simulink library "stb"  (Simulink 8.1)
settings: Solver=ode1  StartTime=0.0  StopTime=Inf  FixedStep=0.001  RelTol=1e-3
PostLoadFcn:
  | , if any(exist('dsrtsu_mdlpostloadfcn', 'file') == [2, 3, 6]), try dsrtsu_mdlpostloadfcn('Execute', bdroot); catch fprintf('Error in PostLoadFcn (dsrtsu_mdlpostloadfcn) for model "%s":\n %s\n', bdroot, lasterr); end, end,
undefined symbols (not defined in the file or in its folder): KACC_ACCDecelReleaseMargin_kph, KACC_ACCDecelStartMargin_kph
libraries: hcu_lib x3
settings Model: DSRTSU_INTERNAL_RTI_VER=450  DSRTSU_INTERNAL_RTI_TYPE=rti1401  RTICANMMDATA=struct('GeneralSetupData',struct('modelroot','D:\ELN150201_TAIWAN\trunk\AdasDragon\software\sw_development\arch\app\acc','generalsettings',struct('filesettings',struct('destfolder',struct('Name','RTICANMM_FILES','Check',1),'buildfolder',struct('Name','.','Check',1),'AbsDestfolder',struct('Name','D:\ELN150201_TAIWAN\trunk\AdasDragon\software\sw_development\arch\app\acc\RTICANMM_FILES'),'AbsBuildfolder',struct('Name','D:\ELN150201_TAIWAN\trunk\AdasDragon\software\sw_development\arch\app\acc'))),'options',struct('addpaths',1,'rmpaths',1,'addtrcexclusion',logical(1),'cannavigator',struct('checkmonitoring',0),'show_usrtrc',0,'use_usrtrc',0),'advanced',struct('options',[1 1 1 1 1 1 1 1 1 1 1 1 1 1 1 1 1 1 1 1 1 1 1 1 1 1 1 1 1 1 1 1 1 1 1 1 1 1 1 1 1 1 1 1 1 1 1 1 1 1 1 1 1 1 1 1 1 1 1 1 1 1 1 1 1 1 1 1 1 1 1 1 1 1 1 1 1 1 1 1 1 1 1 1 1 1 1 1 1 1 1 1 1 1 1 1 1 1 1 1]),'MPSetup',{{}},'modelname','stb','block','stb'))  DSRTSU_INTERNAL_RTIFPGA=40  Creator=AT015555  LastModifiedBy=AT015555

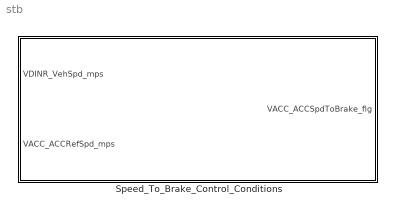
== system stb ==
  Speed_To_Brake_Control_Conditions : Subsystem

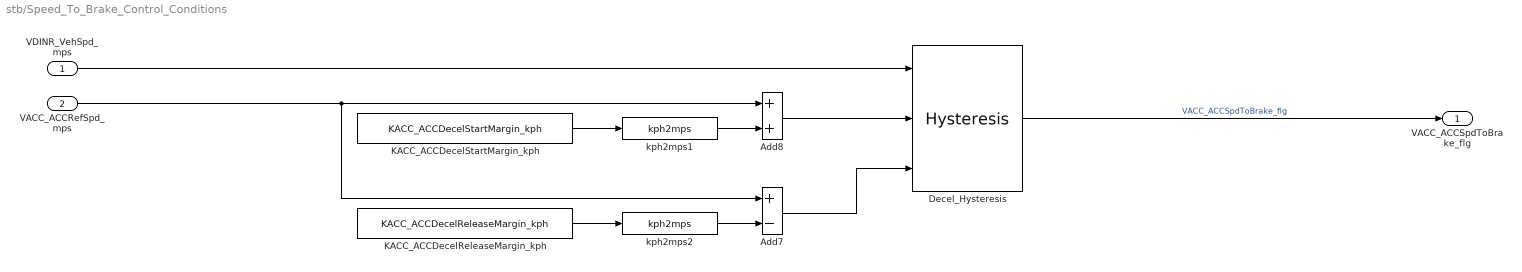
== system stb/Speed_To_Brake_Control_Conditions ==
  VDINR_VehSpd_mps : Inport
  VACC_ACCRefSpd_mps : Inport  Port=2
  Add7 : Sum  Inputs=+-
  Add8 : Sum
  Decel_Hysteresis : hcu_lib/Hysteresis  SystemSampleTime=-1
  KACC_ACCDecelReleaseMargin_kph : Constant  Value=KACC_ACCDecelReleaseMargin_kph  OutDataTypeStr=single
  KACC_ACCDecelStartMargin_kph : Constant  Value=KACC_ACCDecelStartMargin_kph  OutDataTypeStr=single
  kph2mps1 : hcu_lib/kph2mps
  kph2mps2 : hcu_lib/kph2mps
  VACC_ACCSpdToBrake_flg : Outport
  wires:
  kph2mps2/1 -> Add7/2
  kph2mps1/1 -> Add8/2
  Add7/1 -> Decel_Hysteresis/3
  Add8/1 -> Decel_Hysteresis/2
  VDINR_VehSpd_mps/1 -> Decel_Hysteresis/1
  KACC_ACCDecelStartMargin_kph/1 -> kph2mps1/1
  KACC_ACCDecelReleaseMargin_kph/1 -> kph2mps2/1
  Decel_Hysteresis/1 -> VACC_ACCSpdToBrake_flg/1  "VACC_ACCSpdToBrake_flg"
  VACC_ACCRefSpd_mps/1 -> Add7/1, Add8/1
